simulink model "schema_numerique"  (R2024b)
settings: Solver=FixedStepAuto  StartTime=0.0  StopTime=10.0  FixedStep=Ts  RelTol=1e-3
values from neighbouring files (symbols this model uses):
  A = -(C_yf + C_yr) / (m * v_x0)    (= -7.29166666667)    [main_data.m]
  B = (-l_f*C_yf + l_r*C_yr) / (m * v_x0) - v_x0    (= -19.8958333333)    [main_data.m]
  C = (-l_f*C_yf + l_r*C_yr) / (I_zz * v_x0)    (= 0.208333333333)    [main_data.m]
  D = -(l_f^2*C_yf + l_r^2*C_yr) / (I_zz * v_x0)    (= -9.14583333333)    [main_data.m]
  E = C_yf / (m * v_x0)    (= 3.125)    [main_data.m]
  F = (l_f * C_yf) / I_zz    (= 112.5)    [main_data.m]
  I_zz = 120    [main_data.m]
  Ts = 0.001    [main_data.m]
settings Model: Creator=marti  LastModifiedBy=marti

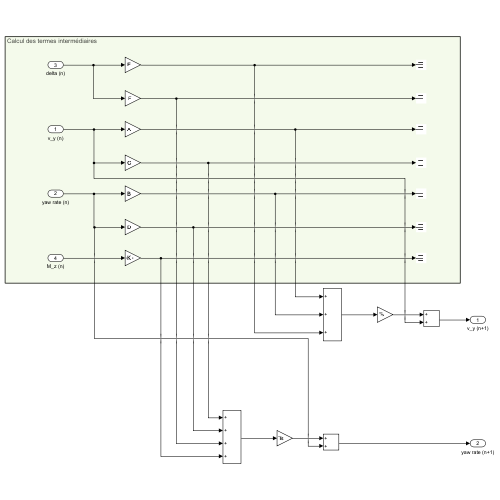
[thumbnail: Simulink's stored preview of the top-level diagram]
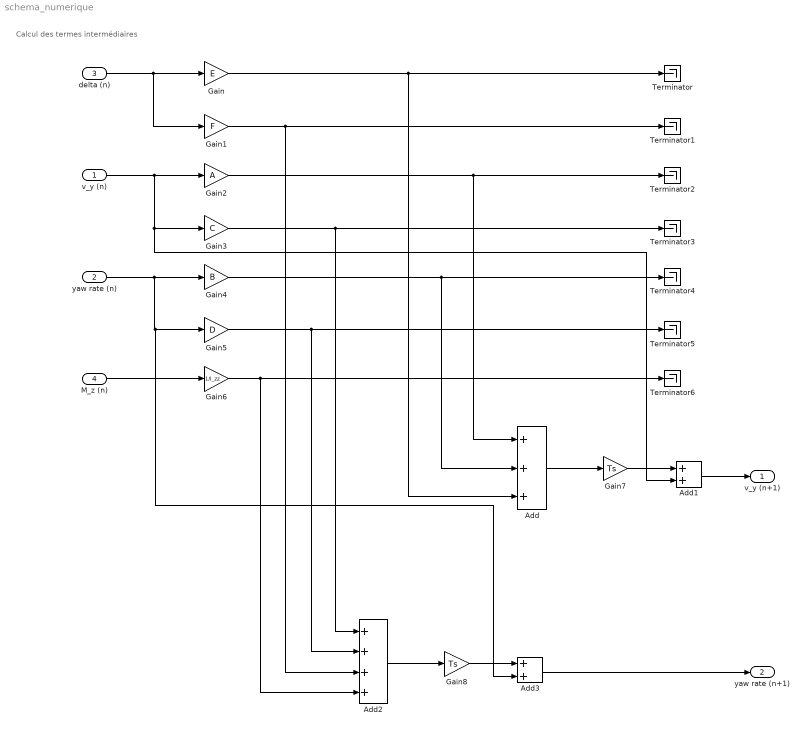
== system schema_numerique ==
  note: Calcul des termes intermédiaires
  v_y (n) : Inport
  yaw rate (n) : Inport  Port=2
  delta (n) : Inport  Port=3
  M_z (n) : Inport  Port=4
  Add : Sum  Inputs=+++
  Add1 : Sum
  Add2 : Sum  Inputs=++++
  Add3 : Sum
  Gain : Gain  Gain=E
  Gain1 : Gain  Gain=F
  Gain2 : Gain  Gain=A
  Gain3 : Gain  Gain=C
  Gain4 : Gain  Gain=B
  Gain5 : Gain  Gain=D
  Gain6 : Gain  Gain=1/I_zz
  Gain7 : Gain  Gain=Ts
  Gain8 : Gain  Gain=Ts
  Terminator{,1..6} (7 alike) : Terminator
  v_y (n+1) : Outport
  yaw rate (n+1) : Outport  Port=2
  wires:
  delta (n)/1 -> Gain1/1, Gain/1
  v_y (n)/1 -> Gain2/1, Add1/2, Gain3/1
  yaw rate (n)/1 -> Add3/2, Gain5/1, Gain4/1
  Gain/1 -> Terminator/1, Add/3
  Gain1/1 -> Add2/3, Terminator1/1
  Gain2/1 -> Terminator2/1, Add/1
  Gain3/1 -> Add2/1, Terminator3/1
  Gain4/1 -> Terminator4/1, Add/2
  Gain5/1 -> Add2/2, Terminator5/1
  Gain6/1 -> Add2/4, Terminator6/1
  M_z (n)/1 -> Gain6/1
  Add/1 -> Gain7/1
  Gain7/1 -> Add1/1
  Gain8/1 -> Add3/1
  Add2/1 -> Gain8/1
  Add1/1 -> v_y (n+1)/1
  Add3/1 -> yaw rate (n+1)/1
